simulink model "synchronous_generator_and_load"  (R2021a)
settings: Solver=VariableStepAuto  StartTime=0.0  StopTime=60  RelTol=1e-3
libraries: spsThreePhaseVIMeasurementLib x3, spsLoadFlowBusLib x3, spsPower3phInstantaneousLib x3, spsMultimeterLib x2, spsThreePhaseSeriesRLCBranchLib x2, spsSynchronousMachinepuStandardLib x1, spsGroundLib x1, spsThreePhaseParallelRLCLoadLib x1, spsThreePhaseSourceLib x1, spsThreePhaseTransformerTwoWindingsLib x1, spspowerguiLib x1
settings Model: Creator=Asus  LastModifiedBy=Asus

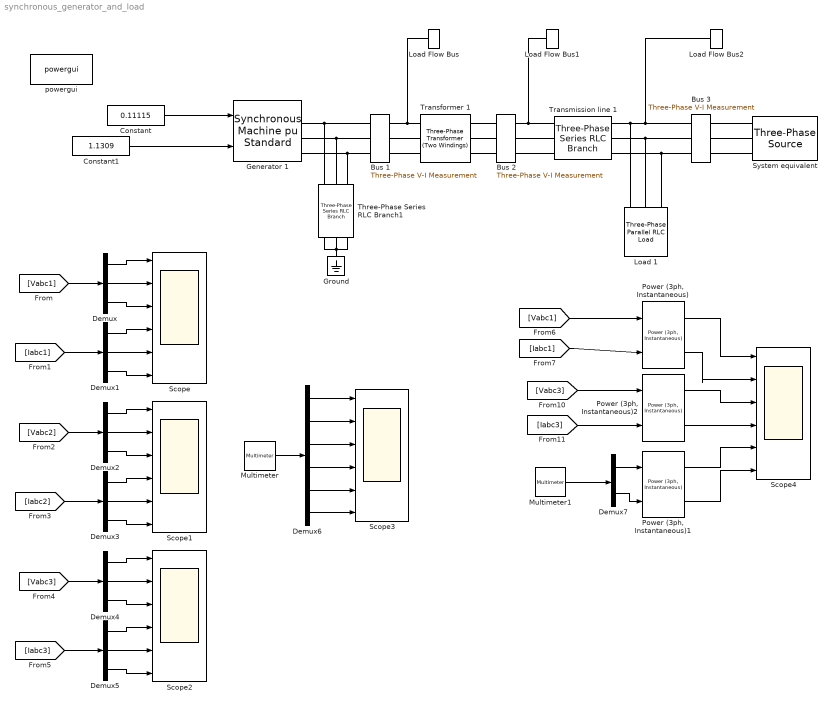
== system synchronous_generator_and_load ==
  Bus 1 : spsThreePhaseVIMeasurementLib/Three-Phase V-I Measurement  VoltageMeasurement=phase-to-ground  SetLabelV=on  LabelV=Vabc1  Vpu=off  VpuLL=off  CurrentMeasurement=yes  SetLabelI=on  LabelI=Iabc1  Ipu=off  Pbase=100e6  Vbase=500e3  OutputType=Complex  PhasorSimulation=off  PSBequivalent=0
  Bus 2 : spsThreePhaseVIMeasurementLib/Three-Phase V-I Measurement  VoltageMeasurement=phase-to-ground  SetLabelV=on  LabelV=Vabc2  Vpu=off  VpuLL=off  CurrentMeasurement=yes  SetLabelI=on  LabelI=Iabc2  Ipu=off  Pbase=100e6  Vbase=500e3  OutputType=Complex  PhasorSimulation=off  PSBequivalent=0
  Bus 3 : spsThreePhaseVIMeasurementLib/Three-Phase V-I Measurement  VoltageMeasurement=phase-to-ground  SetLabelV=on  LabelV=Vabc3  Vpu=off  VpuLL=off  CurrentMeasurement=yes  SetLabelI=on  LabelI=Iabc3  Ipu=off  Pbase=100e6  Vbase=500e3  OutputType=Complex  PhasorSimulation=off  PSBequivalent=0
  Constant : Constant  Value=0.11115
  Constant1 : Constant  Value=1.1309
  Demux{,1..5} (6 alike) : Demux  Outputs=3
  Demux6 : Demux  Outputs=6
  Demux7 : Demux  Outputs=2
  Generator 1 : spsSynchronousMachinepuStandardLib/Synchronous Machine pu Standard  PresetModel=No  MechanicalLoad=Mechanical power Pm  ShowDetailedParameters=on  RotorType=Round  Units=per unit standard parameters  MeasurementBus=off  NominalParameters="[900e+6  20e+3 60]"  Reactances1=[ 1.81, 0.3, 0.25, 1.70, 0.55, 0.25, 0.20 ]  Reactances2=[2.24 0.17 0.12 1.02 0.13 0.08]  dAxisTimeConstants=Open-circuit  qAxisTimeConstants=Open-circuit  TimeConstants1="[ 4.4849  0.0681  0.1  ]"  TimeConstants2=[ 8.0, 0.03, 0.40, 0.05 ]  TimeConstants3="[  4.49  0.0681  0.0513  ]"  TimeConstants4=[ 8.0, 0.03, 0.3371, 0.0295 ]  TimeConstants5=[ 1.01, 0.053, 0.1 ]  TimeConstants6=[8.00, 0.03, 0.40, 0.05 ]  TimeConstants7=[0.012 0.003 0.003]  TimeConstants8=[ 1.3201, 0.0231, 0.3371, 0.0295 ]  StatorResistance=0.0025  Mechanical=[6.50 0.02 1]  PolePairs=20  InitialConditions=[0 -79.1383 0.122505 0.122505 0.122505 -25.2441 -145.244 94.7559 1.13093]  SetSaturation=off  Saturation=[0.6404,0.7127,0.8441,0.9214,0.9956,1.082,1.19,1.316,1.457;0.7,0.7698,0.8872,0.9466,0.9969,1.046,1.1,1.151,1.201]  LoadFlowParameters=[1,0,0,0,0]  TsPowergui=0  TsBlock=-1  IterativeModel=Trapezoidal non iterative  IterativeDiscreteModel=Trapezoidal non iterative  BusType=PQ  Pref=100000000  Qref=50000000  Qmin=-Inf  Qmax=Inf  PLF=0  QLF=0
      settings: SourceProductBaseCode=PS
  Ground : spsGroundLib/Ground  LConnTagsString=a
  Load 1 : spsThreePhaseParallelRLCLoadLib/Three-Phase Parallel RLC Load  LConnTagsString=A|B|C  Configuration=Y (grounded)  NominalVoltage=230e3  Vabc=[1e3 1e3 1e3]  Vabcp=[1e3 1e3 1e3]  NominalFrequency=60  UnbalancedPower=off  ActivePower=200000000  InductivePower=100000000  CapacitivePower=0  Pabc=[10e3 9e3 11e3]  QLabc=[100 90 110]  QCabc=[100 90 110]  Pabcp=[10e3 9e3 11e3]  QLabcp=[100 90 110]  QCabcp=[100 90 110]  Measurements=Branch voltages and currents  LoadType=constant Z
  Load Flow Bus : spsLoadFlowBusLib/Load Flow Bus  LConnTagsString=a  Phases=single  Connectors=on one side  ID=BUS_1  Vbase=20e3  Vref=1  Vangle=0  VLF=1.014  VLFb=1  VLFc=1  angleLF=1.321  angleLFb=0  angleLFc=0
      settings: SourceProductBaseCode=PS
  Load Flow Bus1 : spsLoadFlowBusLib/Load Flow Bus  LConnTagsString=a  Phases=single  Connectors=on one side  ID=BUS_2  Vbase=230e3  Vref=1  Vangle=0  VLF=1.014  VLFb=1  VLFc=1  angleLF=1.318  angleLFb=0  angleLFc=0
      settings: SourceProductBaseCode=PS
  Load Flow Bus2 : spsLoadFlowBusLib/Load Flow Bus  LConnTagsString=a  Phases=single  Connectors=on one side  ID=BUS_3  Vbase=230e3  Vref=1  Vangle=0  VLF=1  VLFb=1  VLFc=1  angleLF=0  angleLFb=0  angleLFc=0
      settings: SourceProductBaseCode=PS
  Multimeter : spsMultimeterLib/Multimeter  PhasorSimulation=off  OutputType=Complex  sel=[1 2 3 4 5 6]  L=6  Gain=[1 1 1 1 1 1]  yselected={'Uag: Load 1','Ubg: Load 1','Ucg: Load 1','Iag: Load 1','Ibg: Load 1','Icg: Load 1'};  PSBOutputType=1  PSBequivalent=0  AxesSetting=[0,0.1,-100,100]  Display=0  SavedBlockNames=-11
  Multimeter1 : spsMultimeterLib/Multimeter  PhasorSimulation=off  OutputType=Complex  sel=[1 2 3 4 5 6]  L=6  Gain=[1 1 1 1 1 1]  yselected={'Uag: Load 1','Ubg: Load 1','Ucg: Load 1','Iag: Load 1','Ibg: Load 1','Icg: Load 1'};  PSBOutputType=1  PSBequivalent=0  AxesSetting=[0,0.1,-100,100]  Display=0  SavedBlockNames=-11
  "Power (3ph, Instantaneous)" : spsPower3phInstantaneousLib/Power (3ph, Instantaneous)
  "Power (3ph, Instantaneous)1" : spsPower3phInstantaneousLib/Power (3ph, Instantaneous)
  "Power (3ph, Instantaneous)2" : spsPower3phInstantaneousLib/Power (3ph, Instantaneous)
  Scope{,1..4} (5 alike) : Scope  NumInputPorts=6
  System equivalent : spsThreePhaseSourceLib/Three-Phase Source  InternalConnection=Yg  VoltagePhases=off  Voltage=(230000)*1.01245  PhaseAngle=1.0342  Voltage_phases=[25e3 25e3 25e3]/sqrt(3)  PhaseAngles_phases=[0 -120 +120]  Frequency=60  NonIdealSource=on  SpecifyImpedance=off  Resistance=1  Inductance=0.026525824  ShortCircuitLevel=100e6  BaseVoltage=230e3  XRratio=7  BusType=swing  Pref=10000  Qref=0  Prefabc=[10e3, 10e3, 10e3]  Qrefabc=[0, 0, 0]  Qmin=-Inf  Qmax=Inf
  Three-Phase Series RLC Branch1 : spsThreePhaseSeriesRLCBranchLib/Three-Phase Series RLC Branch  LConnTagsString=A|B|C  RConnTagsString=A|B|C  BranchType=R  Resistance=1e6  Inductance=1e-3  Capacitance=1e-6  Measurements=None
  Transformer 1 : spsThreePhaseTransformerTwoWindingsLib/Three-Phase Transformer (Two Windings)  Winding1Connection=Yg  Winding2Connection=Yg  CoreType=Three single-phase transformers  SetSaturation=off  Hysteresis=off  DataFile='hysteresis'  SetInitialFlux=off  Measurements=None  UNITS=pu  NominalPower=[ 900e6 , 60 ]  Winding1=[ 20000 , 0 , 0.000198944 ]  Winding2=[ 230000 , 0 , 0.000198944 ]  Rm=500  Lm=500  L0=0.5  Saturation=[ 0,0 ; 0.0024,1.2 ; 1.0,1.52 ]  InitialFluxes=[ 0.8 , -0.8 , 0.7 ]  BreakLoop=off  DiscreteSolver=Trapezoidal iterative  DataType=off  TransfoNumber=1
  Transmission line 1 : spsThreePhaseSeriesRLCBranchLib/Three-Phase Series RLC Branch  LConnTagsString=A|B|C  RConnTagsString=A|B|C  BranchType=RL  Resistance=1.3225  Inductance=0.035080402  Capacitance=1e-6  Measurements=None
  powergui : spspowerguiLib/powergui  Priority=1  SimulationMode=Discrete  SampleTime=50e-6  frequency=60  Iterations=50  frequencyindice=60  Pbase=100e6  ErrMax=1e-4  UnitsV=kV  UnitsW=MW  buscounter=0  FunctionMessages=off  echomessages=off  EnableUseOfTLC=off  CurrentSourceSwitches=off  DisableSnubberDevices=off  DisableRonSwitches=off  DisableVfSwitches=off  DisplayEquations=off  AutomaticDiscreteSolvers=off  SolverType=Tustin/Backward Euler (TBE)  Interpol=off  ExternalGateDelay=off  methode=off  Ts=100  x0status=blocks  SPID=on  SwTol=0  HookPort=off  NonlinearTolerance=1e-4  nMaxIteration=100  ContinueOnMaxIteration=off  RestoreLinks=warning  ResistiveCurrentMeasurement=off  Frange=[0:2:500]  Ylog=off  Xlog=on  ShowGrid=off  save=off  variable=ZData  structure=0  ZoomFFT=off  StartTime=0.0  cycles=1  DisplayStyle=1  fundamental=60  FreqAxis=off  MaxFrequency=1000  frequencyindicesteady=1  RmsSteady=1  display=off
  wires:
  Constant/1 -> Generator 1/1
  Constant1/1 -> Generator 1/2
  [Vabc1] -> Demux/1
  [Iabc1] -> Demux1/1
  Demux/1 -> Scope/1
  Demux/2 -> Scope/2
  Demux/3 -> Scope/3
  Demux1/1 -> Scope/4
  Demux1/2 -> Scope/5
  Demux1/3 -> Scope/6
  [Iabc2] -> Demux3/1
  Demux2/1 -> Scope1/1
  [Vabc2] -> Demux2/1
  Demux3/3 -> Scope1/6
  Demux2/2 -> Scope1/2
  Demux3/2 -> Scope1/5
  Demux2/3 -> Scope1/3
  Demux3/1 -> Scope1/4
  [Iabc3] -> Demux5/1
  Demux4/1 -> Scope2/1
  [Vabc3] -> Demux4/1
  Demux5/3 -> Scope2/6
  Demux4/2 -> Scope2/2
  Demux5/2 -> Scope2/5
  Demux4/3 -> Scope2/3
  Demux5/1 -> Scope2/4
  Demux6/3 -> Scope3/3
  Demux6/1 -> Scope3/1
  Multimeter/1 -> Demux6/1
  Demux6/2 -> Scope3/2
  Demux6/4 -> Scope3/4
  Demux6/5 -> Scope3/5
  Demux6/6 -> Scope3/6
  [Vabc1] -> "Power (3ph, Instantaneous)"/1
  [Iabc1] -> "Power (3ph, Instantaneous)"/2
  [Vabc3] -> "Power (3ph, Instantaneous)2"/1
  [Iabc3] -> "Power (3ph, Instantaneous)2"/2
  "Power (3ph, Instantaneous)"/1 -> Scope4/1
  "Power (3ph, Instantaneous)"/2 -> Scope4/2
  "Power (3ph, Instantaneous)2"/1 -> Scope4/3
  "Power (3ph, Instantaneous)2"/2 -> Scope4/4
  Multimeter1/1 -> Demux7/1
  Demux7/1 -> "Power (3ph, Instantaneous)1"/1
  Demux7/2 -> "Power (3ph, Instantaneous)1"/2
  "Power (3ph, Instantaneous)1"/1 -> Scope4/5
  "Power (3ph, Instantaneous)1"/2 -> Scope4/6
  connections:
  Load Flow Bus/LConn1 -- Bus 1/RConn1 -- Transformer 1/LConn1
  Three-Phase Series RLC Branch1/LConn2 -- Bus 1/LConn2 -- Generator 1/RConn2
  Three-Phase Series RLC Branch1/LConn3 -- Bus 1/LConn3 -- Generator 1/RConn3
  Load Flow Bus1/LConn1 -- Bus 2/RConn1 -- Transmission line 1/LConn1
  Transmission line 1/RConn3 -- Bus 3/RConn3 -- Load 1/LConn3
  Transmission line 1/RConn2 -- Bus 3/RConn2 -- Load 1/LConn2
  Load 1/LConn1 -- Bus 3/RConn1 -- Load Flow Bus2/LConn1 -- Transmission line 1/RConn1
  Ground/LConn1 -- Three-Phase Series RLC Branch1/RConn1 -- Three-Phase Series RLC Branch1/RConn2 -- Three-Phase Series RLC Branch1/RConn3
  Generator 1/RConn1 -- Bus 1/LConn1 -- Three-Phase Series RLC Branch1/LConn1
  Bus 1/RConn3 -- Transformer 1/LConn3
  Bus 1/RConn2 -- Transformer 1/LConn2
  Bus 2/RConn2 -- Transmission line 1/LConn2
  Bus 2/RConn3 -- Transmission line 1/LConn3
  Bus 2/LConn3 -- Transformer 1/RConn3
  Bus 2/LConn1 -- Transformer 1/RConn1
  Bus 2/LConn2 -- Transformer 1/RConn2
  Bus 3/LConn1 -- System equivalent/RConn1
  Bus 3/LConn2 -- System equivalent/RConn2
  Bus 3/LConn3 -- System equivalent/RConn3
